simulink model "InvertedPendulumWithLinealization_s"  (R2017a)
settings: Solver=VariableStepAuto  StartTime=0.0  StopTime=10000  FixedStep=1  RelTol=1e-3
libraries: powerlib_meascontrol x1
settings Model: Creator=aposad31  LastModifiedBy=Asus

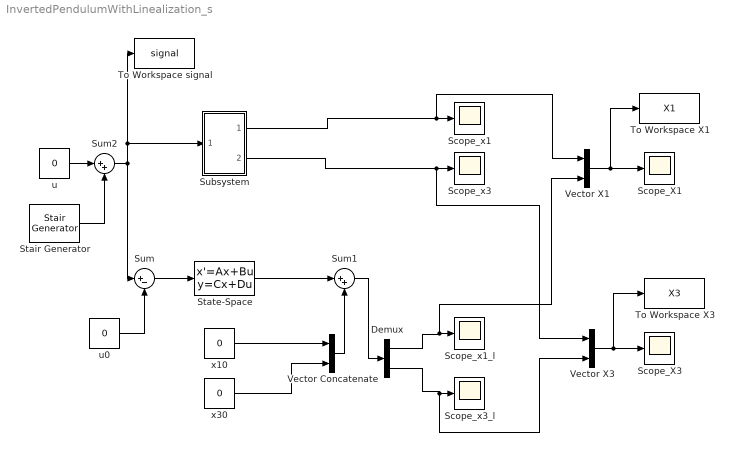
== system InvertedPendulumWithLinealization_s ==
  Demux : Demux  Outputs=2
  Scope_X1 : Scope
  Scope_X3 : Scope
  Scope_x1 : Scope
  Scope_x1_l : Scope
  Scope_x3 : Scope
  Scope_x3_l : Scope
  Stair Generator : powerlib_meascontrol/Pulse & Signal Generators/Stair Generator  t=T  e=Step  Ts=0
      settings: SourceProductName=Simscape Power Systems
  State-Space : StateSpace  A=[0 1 0 0; 0 -2/11 147/55 0; 0 0 0 1; 0 5/11 -343/11 0]  B=[0; 20/11; 0; -50/11]  C=[1 0 0 0; 0 0 1 0]  D=[0; 0]  X0=0
  Subsystem : Subsystem  mask{M=0.5, m_p=0.2, b=0.1, L=0.3, I=0.006, g=9.8, dx10=0, dx20=0, dx30=0, dx40=0}
      mask prompts: m_p "m"
      mask TypeOptions M: M/Value
      mask TypeOptions m_p: m/Value
      mask TypeOptions b: b/Value
      mask TypeOptions L: L/Value
      mask TypeOptions I: I/Value
      mask TypeOptions g: g/Value
      mask TypeOptions dx10: dx1/InitialCondition
      mask TypeOptions dx20: dx2/InitialCondition
      mask TypeOptions dx30: dx3/InitialCondition
      mask TypeOptions dx40: dx4/InitialCondition
  Sum : Sum  Inputs=|+-
  Sum1 : Sum  Inputs=|++
  Sum2 : Sum  Inputs=|++
  To Workspace X1 : ToWorkspace  VariableName=X1  SaveFormat=Timeseries  SampleTime=-1
  To Workspace X3 : ToWorkspace  VariableName=X3  SaveFormat=Timeseries  SampleTime=-1
  To Workspace signal : ToWorkspace  VariableName=signal  SaveFormat=Timeseries  SampleTime=-1
  Vector Concatenate : Concatenate
  Vector X1 : Concatenate
  Vector X3 : Concatenate
  u : Constant  Value=0
  u0 : Constant  Value=0
  x10 : Constant  Value=0
  x30 : Constant  Value=0
  wires:
  Sum/1 -> State-Space/1
  u0/1 -> Sum/2
  State-Space/1 -> Sum1/1
  Vector Concatenate/1 -> Sum1/2
  x30/1 -> Vector Concatenate/2
  x10/1 -> Vector Concatenate/1
  Sum1/1 -> Demux/1
  Subsystem/1(Out1) -> Vector X1/1, Scope_x1/1
  Subsystem/2(Out2) -> Vector X3/1, Scope_x3/1
  Demux/1 -> Vector X1/2, Scope_x1_l/1
  Demux/2 -> Vector X3/2, Scope_x3_l/1
  u/1 -> Sum2/1
  Stair Generator/1 -> Sum2/2
  Vector X3/1 -> To Workspace X3/1, Scope_X3/1
  Vector X1/1 -> To Workspace X1/1, Scope_X1/1
  Sum2/1 -> Subsystem/1(In3), To Workspace signal/1, Sum/1

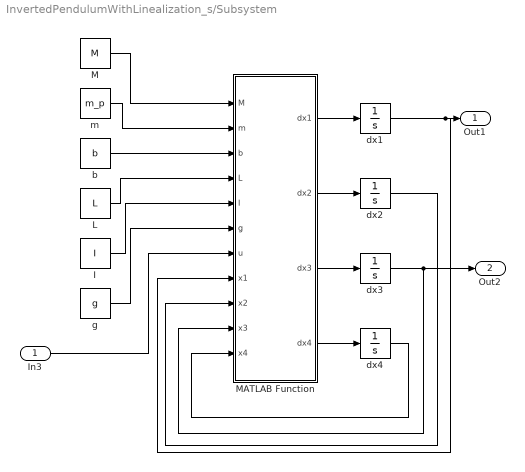
== system InvertedPendulumWithLinealization_s/Subsystem ==
  In3 : Inport
  I : Constant  Value=I
  L : Constant  Value=L
  M : Constant  Value=M
  MATLAB Function : MATLAB Function  TreatAsAtomicUnit=on
  b : Constant  Value=b
  dx1 : Integrator  InitialCondition=dx10
  dx2 : Integrator  InitialCondition=dx20
  dx3 : Integrator  InitialCondition=dx30
  dx4 : Integrator  InitialCondition=dx40
  g : Constant  Value=g
  m : Constant  Value=m_p
  Out1 : Outport
  Out2 : Outport  Port=2
  wires:
  dx1/1 -> MATLAB Function/8(x1), Out1/1
  MATLAB Function/2(dx2) -> dx2/1
  In3/1 -> MATLAB Function/7(u)
  m/1 -> MATLAB Function/2(m)
  MATLAB Function/1(dx1) -> dx1/1
  dx3/1 -> MATLAB Function/10(x3), Out2/1
  dx4/1 -> MATLAB Function/11(x4)
  MATLAB Function/3(dx3) -> dx3/1
  M/1 -> MATLAB Function/1(M)
  b/1 -> MATLAB Function/3(b)
  MATLAB Function/4(dx4) -> dx4/1
  dx2/1 -> MATLAB Function/9(x2)
  g/1 -> MATLAB Function/6(g)
  L/1 -> MATLAB Function/4(L)
  I/1 -> MATLAB Function/5(I)

== matlab function InvertedPendulumWithLinealization_s/Subsystem/MATLAB Function ==
  data: M input; m input; b input; L input; I input; g input; u input; dx1 output; x1 input; x2 input; x3 input; x4 input; dx2 output; dx3 output; dx4 output
function [dx1, dx2, dx3, dx4] = fcn(M, m, b, L, I, g, u, x1, x2, x3, x4)
    denominator = (M+m)*(I+m*L^2)-m^2*L^2*cos(x3)^2;
    dx1 = x2;
    dx2 = ((I+m*L^2)*(u-b*x2+m*L*x4^2*sin(x3))+m^2*L^2*g*sin(x3)*cos(x3))/denominator;
    dx3 = x4;
    dx4 = (-m*L*u*cos(x3)+m*L*b*x2*cos(x3)-m^2*L^2*x4^2*sin(x3)*cos(x3)-(M+m)*m*g*L*sin(x3))/denominator;
end
